simulink model "Continuous2_2018a"  (R2018a)
settings: Solver=VariableStepAuto  StartTime=0.0  StopTime=1.5  FixedStep=0.1  RelTol=1e-3  EnableMultiTasking=on
settings Model: Creator=BEAR  LastModifiedBy=bzhan
settings SolverCC: AutoInsertRateTranBlk=on
settings DataIOCC: LimitDataPoints=on
settings OptimizationCC: LifeSpan=inf
settings DebuggingCC: AllowSymbolicDim=off  SFUnexpectedBacktrackingDiag=warning  SFNoUnconditionalDefaultTransitionDiag=warning  SFExecutionAtInitializationDiag=none
settings CodeAppCC: StateflowObjectComments=on
settings GRTTargetCC: TargetLangStandard=C89/C90 (ANSI)
settings ConfigComp: CovMetricSettings=dw  CovHtmlReporting=on  CovSaveCumulativeToWorkspaceVar=on  CovSaveSingleToWorkspaceVar=on  CovShowResultsExplorer=off  CovExternalEMLEnable=off  CovSFcnEnable=off

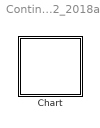
== system Continuous2_2018a ==
  Chart : Stateflow chart  TreatAsAtomicUnit=on

== stateflow chart Continuous2_2018a/Chart ==
  settings: updateMethod=CONTINUOUS
  state A
    en: f("enA")
    du: x_dot=y; y_dot=-x;
    ex: f("exA")
  state B
    en: f("enB"); x=0;
    du: x_dot=1;
    state B1
      en: f("enB1")
    (default) -> B1
  (default) -> A : {x=0;y=1;}
  A -> B1 : [x >= 0.5]{f("conAB1")}/{f("tranAB1")}
  B -> B : [x>=1]
  data: s function_input; y local double; x local double
  data y settings: updateMethod=SF_CONTINUOUS_TIME_DATA
  data x settings: updateMethod=SF_CONTINUOUS_TIME_DATA
  function f(s):
    | function f(s)
    |     fprintf(s+' %.3f %.3f\n', x, y);
